simulink model "Longitudinal_Stability_Model"  (R2013a)
settings: Solver=ode45  StartTime=0.0  StopTime=60  RelTol=1e-6
values from neighbouring files (symbols this model uses):
  DEN = [12.3699,81.5615,13.1192,28.2955,0.002364]    [Controller_Design.m]
  k = -K    [Controller_Design.m]
  NUM = [-61.877,-284.018,-54.0823,-0.00260016,0]    [Controller_Design.m]
settings Model: Creator=Willdog  LastModifiedBy=Willdog

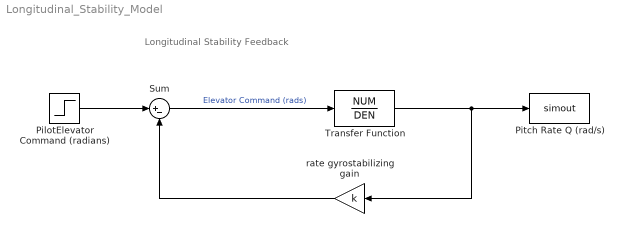
== system Longitudinal_Stability_Model ==
  note: Longitudinal Stability Feedback
  PilotElevator Command (radians) : Step  After=0.03  SampleTime=0
  Pitch Rate Q (rad/s) : ToWorkspace  VariableName=simout  SampleTime=-1  SaveFormat=Timeseries
  Sum : Sum  Inputs=|+-
  Transfer Function : TransferFcn  Numerator=NUM  Denominator=DEN
  rate gyrostabilizing gain : Gain  Gain=k
  wires:
  Sum/1 -> Transfer Function/1  "Elevator Command (rads)"
  rate gyrostabilizing gain/1 -> Sum/2
  Transfer Function/1 -> rate gyrostabilizing gain/1, Pitch Rate Q (rad/s)/1
  PilotElevator Command (radians)/1 -> Sum/1
